simulink model "TaskServiceBase_FSM_revC_MDL"  (Simulink 8.6)
settings: Solver=ode4  StartTime=0.0  StopTime=inf  FixedStep=.01  RelTol=1e-3
settings Model: Creator=elliocm  LastModifiedBy=elliocm
settings DataIOCC: SaveFormat=Dataset  SignalLoggingSaveFormat=Dataset
settings OptimizationCC: ExpressionDepthLimit=128
settings DebuggingCC: UnderspecifiedInitializationDetection=Simplified  MergeDetectMultiDrivingBlocksExec=error  SolverPrmCheckMsg=none  FcnCallInpInsideContextMsg=EnableAllAsError  StateNameClashWarn=none
settings HardwareCC: ProdBitPerPointer=64  ProdLargestAtomicFloat=Float  ProdIntDivRoundTo=Zero  ProdEndianess=LittleEndian  ProdWordSize=64  ProdHWDeviceType=Intel->x86-64 (Windows64)
settings GRTTargetCC: GeneratePreprocessorConditionals=Use local settings  CombineOutputUpdateFcns=on  GRTInterface=off
settings ConfigComp: CovModelRefEnable=off

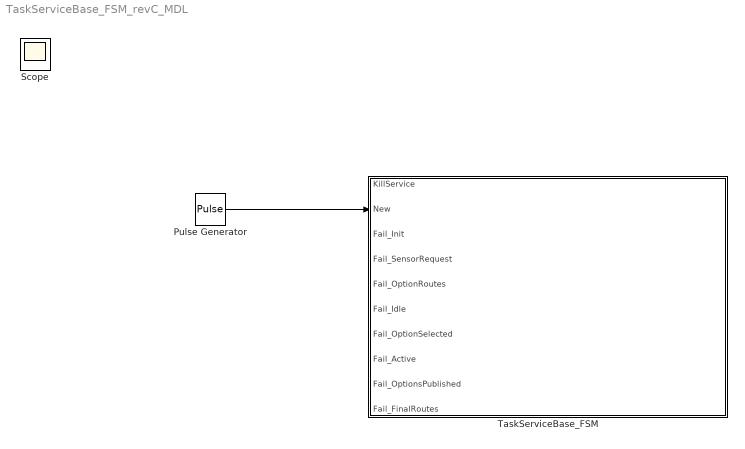
== system TaskServiceBase_FSM_revC_MDL ==
  Pulse Generator : DiscretePulseGenerator  PulseType=Time based  Period=10  PulseWidth=5
  TaskServiceBase_FSM : Stateflow chart  RequirementInfo="{}  %GIDa_69d87331_3a4c_4800_b6a9_49c4bb62fd68"  TreatAsAtomicUnit=on
  Scope : Scope
  wires:
  Pulse Generator/1 -> TaskServiceBase_FSM/2(New)

== stateflow chart TaskServiceBase_FSM ==
  note: CreateNewService
  state TaskServiceBase
    entry: TaskServiceOn = 1
    state Idle
      entry: state = 2
      note: Idle : This represents the state of a Task after initialization, but before any requests have been made that include the Task . UniqueAutomationRequest messages trigger a transition from this state into the SensorRequest state.
          | guarantee "[Not originally specified: in the idle state, once an automation request
          | is recieved that is present in the set of expected task IDs, send a SensorFootprintRequests_out]"
          |
          | guarantee "UniqueAutomationRequestÂ messages trigger a transition from the idle state into theÂ SensorRequestÂ state.
          | When aÂ TaskÂ is notified of its inclusion (by noting the presence of its ID in theÂ TasksÂ list of anÂ
          | UniqueAutomationRequestÂ message), it can request calculations that pertain to the sensors onboard the vehicles
          | that are also included in theÂ UniqueAutomationRequestÂ message.
          | [ASSUMPTION: calculations requests are assumed to mean SensorFootprintRequests_in]"
      state Idle_Request
        entry: SensorFootprintRequests_out = 0
      note: UniqueAutomationRequest (2ms)
          | (Consider Random Fail on Receipt)
      state Idle_Success
        entry: SensorFootprintRequests_out = 1
      (default) -> Idle_Request
      Idle_Request -> (junction 58)
      (junction 58) -> Idle_Success : [after(2,msec) && ~Fail_Idle]
    state SensorRequest
      entry: state = 3
      note: SensorRequest : When a Task is notified of its inclusion (by noting the presence of its ID in the Tasks list of an UniqueAutomationRequest message), it can request calculations that pertain to the sensors onboard the vehicles that are also included in the UniqueAutomationRequest message. While waiting for a response from the SensorManagerService , a Task is in the SensorRequest state and will remain so until the response from the SensorManagerService is received.
          | guarantee "[Not originally specified: in the SENSOR_REQUEST state, if the expected SensorFootprintResponse_in is received send a RouteRequest_out]"
          |
          | guarantee "[IMPLIED: in the SensorRequest state] After theÂ SensorManagerServiceÂ has replied with the appropriate sensor calculations [IMPLIED: the service will then be in OptionRoutes state]" :
      state SensorRequest_Init
        entry: RouteRequest_out = 0
      note: Processing Time for SensorManagerService
          | (Consider Random Fail on Receipt)
      state SensorRequest_Success
        entry: RouteRequest_out = 1
      (default) -> SensorRequest_Init
      SensorRequest_Init -> (junction 62)
      (junction 62) -> SensorRequest_Success : [after(3,msec) && ~Fail_SensorRequest]
    state Init
      entry: state = 1
      note: Init : This is the state that all Tasks start in and remain until all internal initialization is complete.
          | For example, a Task may need to load complex terrain or weather data upon creation and will
          | require some (possibly significant) start-up time. When a Task has completed its internal initialization,
          | it must report transition from this state via the TaskInitialized message.
          |
          | guarantee "all tasks remain in init until all internal initialization is complete, transitioning to idle after.
          | When aÂ TaskÂ has completed its internal initialization, it must report transition from this state
          | via theÂ TaskInitializedÂ message."
      state Init_Request
        entry: init_complete = 0
        TaskInitialized_out = 0
      state Init_Success
        entry: init_complete = 1
        TaskInitialized_out = 1
      note: Simple Delay
          | (Consider Random Fail on TaskInit)
      (default) -> Init_Request
      Init_Request -> (junction 66)
      (junction 66) -> Init_Success : [after(100,msec) && ~Fail_Init]
    state OptionRoutes
      entry: state = 4
      note: OptionRoutes : After the SensorManagerService has replied with the appropriate sensor calculations, the Task can request waypoints from the RouteAggregatorService that carry out the on- Task goals. For example, an AreaSearchTask can request routes from key surveillance positions that ensure sensor coverage of the entire area. The Task remains in the OptionRoutes state until the RouteAggregatorService replies.
          | guarantee "[Not originally specified: if in the OPTION_ROUTES state and an expected RouteResponse_in is received send an event(TaskPlanOptions_out)]"
          |
          | guarantee "TheÂ TaskÂ remains in theÂ OptionRoutesÂ state until theÂ RouteAggregatorServiceÂ replies.
          | When routes are returned [IMPLIED: from the route aggregator service the service will be in the OPTIONS_PUBLISHED state]
          | [ASSUMPTION: the replies are assumed to be RoutePlanResponse_in]"
      state OptionRoutes_Init
        entry: TaskPlanOptions_out = 0
      note: Processing Time for RouteAggregatorService - COLLECTOR ROLE
          | (Consider Random Fail on Receipt)
      state OptionRoutes_Success
        entry: TaskPlanOptions_out = 1
      (default) -> OptionRoutes_Init
      OptionRoutes_Init -> (junction 70)
      (junction 70) -> OptionRoutes_Success : [after(150,msec) && ~Fail_OptionRoutes]
    state Active
      entry: state = 8
      note: Active : If the Task is in the OptionSelected state and an EntityState message is received which includes the Task ID in the AssociatedTaskList , then the Task switches to the Active state and is allowed to publish new waypoints and sensor commands at will. A Task remains in the Active state until a subsequent EntityState message does not list the Task ID in its AssociatedTaskList . At which point, a transition to Completed is made. Note that a Task can reliquish control indirectly by sending the vehicle to a waypoint not tagged with its own ID. Likewise, it can maintain control indefinitely by ensuring that the vehicle only ever go to a waypoint that includes its ID. If a UniqueAutomationRequest message that includes this Task ID is received in the Active state, it transitions to the Completed state.
      state Active_Init
        entry: TaskComplete_out = 0
      note: Simple Delay
          | (Consider Closed Loop on Task Execution)
      state Active_Success
        entry: TaskComplete_out = 1
        %exit: EntityState_in = 0
        %exit: entity_state_task_id_present = 1
      state Active_NewUniqueAutomationRequest
        entry: TaskComplete_out = 1
        %exit: EntityState_in = 0
        %exit: entity_state_task_id_present = 1
      (default) -> Active_Init
      Active_Init -> (junction 74)
      (junction 74) -> (junction 75) [order 1] : [after(1500,msec) && ~Fail_Active]
      (junction 74) -> (junction 76) [order 2]
      (junction 75) -> Active_Success
      (junction 76) -> Active_NewUniqueAutomationRequest : [New]
    state OptionSelected
      entry: state = 7
      note: OptionSelected : When the final waypoints are returned from the RouteAggregatorService , the Task publishes a complete TaskImplementationResponse message. A Task will remain in this state until an EntityState message includes this Task ID in its AssociatedTaskList . If during this state, a subsequent UniqueAutomationRequest is made, the Task returns to the SensorRequest state and immediately attempts to fulfill the requirements of the new UniqueAutomationRequest . This behavior implies that a Task can only be part of a single AutomationRequest and subsequent requests always override previous requests.
      state OptionSelected_Init
        entry: SensorFootprintRequests_out = 0
        entry: EntityState_in = 0 % req'd to suppress SF bug
        entry: entity_state_task_id_present = 0 % ditto
      note: Variable Delay a function of AREA Search Parameters
          | MATRIX OPTIMIZATION here
          | Discussion w/ Derek
          | ROUTE COLLECTOR
      state OptionSelected_NewUniqueAutomationRequest
        entry: SensorFootprintRequests_out = 1
        entry: EntityState_in = 0
        entry: entity_state_task_id_present = 0
      state OptionSelected_Success
        entry: EntityState_in = 1
        entry: entity_state_task_id_present = 1
        entry: SensorFootprintRequests_out = 0
      (default) -> OptionSelected_Init
      OptionSelected_Init -> (junction 83)
      (junction 83) -> OptionSelected_Success [order 2] : [~Fail_OptionSelected && ~New]
      (junction 83) -> OptionSelected_NewUniqueAutomationRequest [order 1] : [New]
    state OptionsPublished
      entry: state = 5
      note: OptionsPublished : When routes are returned to the Task , it will utilize all route and sensor information to identify and publish the applicable TaskOptions . The determination of TaskOptions is key to overall mission performance and vehicle behavior. It is from this list of options that the assignment will select in order to perform this particular Task . After publication of the options, a Task waits in the OptionsPublished state until the TaskImplementationRequest message is received, whereupon it switches to FinalRoutes .
      state OptionsPublished_Init
        entry: RouteRequest_out = 0
      note: TaskImplementationRequest (2ms)
          | (Consider Random Fail on Receipt)
      state OptionsPublished_Success
        entry: RouteRequest_out = 1
      (default) -> OptionsPublished_Init
      OptionsPublished_Init -> (junction 88)
      (junction 88) -> OptionsPublished_Success : [after(2,msec) && ~Fail_OptionsPublished]
    state FinalRoutes
      entry: state = 6
      note: FinalRoutes : Upon reception of a TaskImplementationRequest , a Task is informed of the option that was selected by the assignment service. At this point, a Task must create the final set of waypoints that include both enroute and on-task waypoints from the specified vehicle location. The Task is required to create the enroute waypoints since a route refinement is possible, taking advantage of the concrete prior position of the selected vehicle. The Task remains in the FinalRoutes state until the route request is fulfilled by the RouteAggregatorService .
      state FinalRoutes_Init
        entry: TaskImplementationResponse_out = 0
      note: Processing Time for RouteAggregatorService - AGGREGATOR ROLE
          | (Consider Random Fail on Receipt)
      state FinalRoutes_Success
        entry: TaskImplementationResponse_out = 1
      (default) -> FinalRoutes_Init
      FinalRoutes_Init -> (junction 92)
      (junction 92) -> FinalRoutes_Success : [after(3,msec) && ~Fail_FinalRoutes]
    Init -> Idle : [init_complete && TaskInitialized_out]
    Idle -> SensorRequest : [SensorFootprintRequests_out]
    OptionSelected -> SensorRequest [order 1] : [SensorFootprintRequests_out]
    SensorRequest -> OptionRoutes : [RouteRequest_out]
    (default) -> Init
    Active -> Idle : [TaskComplete_out]
    OptionSelected -> Active [order 2] : [EntityState_in && entity_state_task_id_present]
    OptionRoutes -> OptionsPublished : [TaskPlanOptions_out]
    FinalRoutes -> OptionSelected : [TaskImplementationResponse_out]
    OptionsPublished -> FinalRoutes : [RouteRequest_out]
  state TaskServiceOff
    entry: TaskServiceOn = 0
  (default) -> TaskServiceBase
  TaskServiceBase -> TaskServiceOff : [KillService]
  data: state local double; init_complete local double; i local double; TaskInitialized_out local double; SensorFootprintRequests_out local double; RouteRequest_out local double; TaskPlanOptions_out local double; EntityState_in local double; entity_state_task_id_present local double; TaskComplete_out local double; TaskImplementationResponse_out local double; KillService input double; TaskServiceOn local double; New input double; Fail_Init input double; Fail_SensorRequest input double; Fail_OptionRoutes input double; Fail_Idle input double; Fail_OptionSelected input double; Fail_Active input double; Fail_OptionsPublished input double; Fail_FinalRoutes input double
